simulink model "MPC"  (R2024a)
settings: Solver=ode4  StartTime=0.0  StopTime=5  FixedStep=1e-6  RelTol=1e-3
PreLoadFcn:
  | Rs=0.02;
  | Ls=0.4;
  | Sm=0.2205;
  | p=4;
  | J=0.006;
  | B=0;
  | f=60;
libraries: slpidlib x1
settings Model: Creator=Windows10  LastModifiedBy=anugr
settings SolverCC: AlgebraicLoopSolver=TrustRegion
settings DataIOCC: ReturnWorkspaceOutputs=off
settings DebuggingCC: UnconnectedInputMsg=warning  UnconnectedOutputMsg=warning  UnconnectedLineMsg=warning  UnderSpecifiedDimensionMsg=warning
settings ModelReferenceCC: EnableRefExpFcnMdlSchedulingChecks=on
settings RTWCC: GPUComputeCapability=3.5

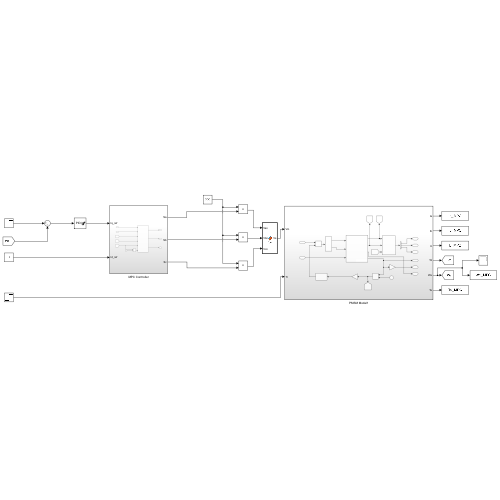
[thumbnail: Simulink's stored preview of the top-level diagram]
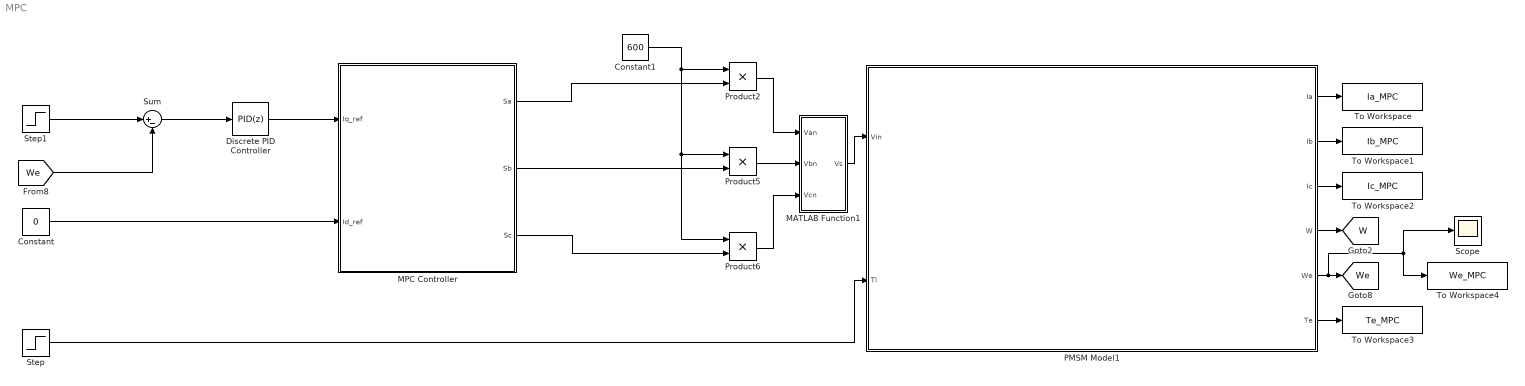
== system MPC ==
  Constant : Constant  Value=0
  Constant1 : Constant  Value=600
  Discrete PID Controller : slpidlib/PID Controller  Controller=PID  Form=Parallel  TimeDomain=Discrete-time  UseExternalTs=off  SampleTime=-1  IntegratorMethod=Forward Euler  FilterMethod=Forward Euler  ControllerParametersSource=internal  P=10  I=1  UseKiTs=off  D=1  UseExternalDerivativeSource=off  N=100  UseFilter=off  TunerSelectOption=Transfer Function Based (PID Tuner App)  InitialConditionSource=internal  InitialConditionForIntegrator=0  InitialConditionForFilter=0  DifferentiatorICPrevScaledInput=0  ExternalReset=none  TrackingMode=off  Kt=1  LimitOutput=on  SatLimitsSource=internal  UpperSaturationLimit=90  LowerSaturationLimit=-90  LinearizeAsGain=on  AntiWindupMode=clamping  Kb=1  LimitIntegrator=off  UpperIntegratorSaturationLimit=inf  LowerIntegratorSaturationLimit=-inf  POutMin=[]  POutMax=[]  IOutMin=[]  IOutMax=[]  DOutMin=[]  DOutMax=[]  NOutMin=[]  NOutMax=[]  SumOutMin=[]  SumOutMax=[]  SaturationOutMin=[]  SaturationOutMax=[]  PParamMin=[]  PParamMax=[]  IParamMin=[]  IParamMax=[]  DParamMin=[]  DParamMax=[]  NParamMin=[]  NParamMax=[]  KbParamMin=[]  KbParamMax=[]  KtParamMin=[]  KtParamMax=[]  KbOutMin=[]  KbOutMax=[]  KtOutMin=[]  KtOutMax=[]  IntegratorOutMin=[]  IntegratorOutMax=[]  FilterOutMin=[]  FilterOutMax=[]  SumI1OutMin=[]  SumI1OutMax=[]  SumI2OutMin=[]  SumI2OutMax=[]  SumI3OutMin=[]  SumI3OutMax=[]  SumI4OutMin=[]  SumI4OutMax=[]  SumDOutMin=[]  SumDOutMax=[]  DifferentiatorOutMin=[]  DifferentiatorOutMax=[]  FilterDiffOutCoefMin=[]  FilterDiffOutCoefMax=[]  ReciprocalOutMin=[]  ReciprocalOutMax=[]  SumDenOutMin=[]  SumDenOutMax=[]  SumNumOutMin=[]  SumNumOutMax=[]  DivideOutMin=[]  DivideOutMax=[]  UdiffTsProdOutMin=[]  UdiffTsProdOutMax=[]  NTsProdOutMin=[]  NTsProdOutMax=[]  UintegralTsProdOutMin=[]  UintegralTsProdOutMax=[]  UngainTsProdOutMin=[]  UngainTsProdOutMax=[]  ClampingZeroOutDataTypeStr=Inherit: Inherit via back propagation  ClampingZeroOutMin=[]  ClampingZeroOutMax=[]  FilterDenConstantOutDataTypeStr=Inherit: Inherit via back propagation  FilterDenConstantOutMin=[]  FilterDenConstantOutMax=[]  PCopyOutDataTypeStr=Inherit: Inherit via back propagation  PCopyOutMin=[]  PCopyOutMax=[]  NCopyOutDataTypeStr=Inherit: Inherit via back propagation  NCopyOutMin=[]  NCopyOutMax=[]  IntegratorContinuousStateAttributes=''  IntegratorStateMustResolveToSignalObject=off  IntegratorRTWStateStorageClass=Auto  FilterContinuousStateAttributes=''  FilterStateMustResolveToSignalObject=off  FilterRTWStateStorageClass=Auto  ParallelPVariant=InternalParameters  IdealPVariant=Disabled  IVariant=InternalParameters  DVariant=InternalParameters  IntegratorVariant=Discrete  SatVariant=Enabled  AWVariant=DiscClampingParallel  PCopyVariant=Disabled  TRVariant=Disabled  FdbkBlocksVariant=Forward  IdealPFdbkVariant=Disabled  SatFdbkVariant=Disabled  DerivativeFilterVariant=Differentiator  NVariant=Passthrough  NCopyVariant=Disabled_SignalSpec  FilterICVariant=InternalICsDifferentiator  IntegratorICVariant=InternalICs  ExternalResetVariant=Disabled  TRSumVariant=Passthrough  SumFdbkVariant=Disabled  SumVariant=Sum_PID  TsampFilterVariant=InternalTs  TsampNgainVariant=Passthrough  TsampIntegralVariant=Disabled_SignalSpec  ExternalSaturationOutDataTypeStr=Inherit: Same as second input  DerivativeSourceVariant=ErrorSignal
  MATLAB Function1 : MATLAB Function  TreatAsAtomicUnit=on
  MPC Controller : Subsystem
  PMSM Model1 : Subsystem
  Product2 : Product
  Product5 : Product
  Product6 : Product
  Scope : Scope
  Step : Step  Time=2.5  After=5  SampleTime=0
  Step1 : Step  Time=2  Before=300  After=800  SampleTime=0
  Sum : Sum  Inputs=|+-
  To Workspace : ToWorkspace  VariableName=Ia_MPC  SaveFormat=Timeseries  SampleTime=-1
  To Workspace1 : ToWorkspace  VariableName=Ib_MPC  SaveFormat=Timeseries  SampleTime=-1
  To Workspace2 : ToWorkspace  VariableName=Ic_MPC  SaveFormat=Timeseries  SampleTime=-1
  To Workspace3 : ToWorkspace  VariableName=Te_MPC  SaveFormat=Timeseries  SampleTime=-1
  To Workspace4 : ToWorkspace  VariableName=We_MPC  SaveFormat=Timeseries  SampleTime=-1
  tag scope: W=global, We=global
  wires:
  Sum/1 -> Discrete PID Controller/1
  [We] -> Sum/2
  Step1/1 -> Sum/1
  Discrete PID Controller/1 -> MPC Controller/1(Iq_ref)
  Step/1 -> PMSM Model1/2(Tl)
  Constant/1 -> MPC Controller/2(Id_ref)
  PMSM Model1/1(Ia) -> To Workspace/1
  PMSM Model1/2(Ib) -> To Workspace1/1
  MATLAB Function1/1(Vs) -> PMSM Model1/1(Vin)
  Constant1/1 -> Product5/1, Product6/1, Product2/1
  Product6/1 -> MATLAB Function1/3(Vcn)
  Product2/1 -> MATLAB Function1/1(Van)
  PMSM Model1/5(We) -> Scope/1, To Workspace4/1, [We]
  PMSM Model1/3(Ic) -> To Workspace2/1
  PMSM Model1/4(W) -> [W]
  Product5/1 -> MATLAB Function1/2(Vbn)
  PMSM Model1/6(Te) -> To Workspace3/1
  MPC Controller/3(Sc) -> Product6/2
  MPC Controller/1(Sa) -> Product2/2
  MPC Controller/2(Sb) -> Product5/2

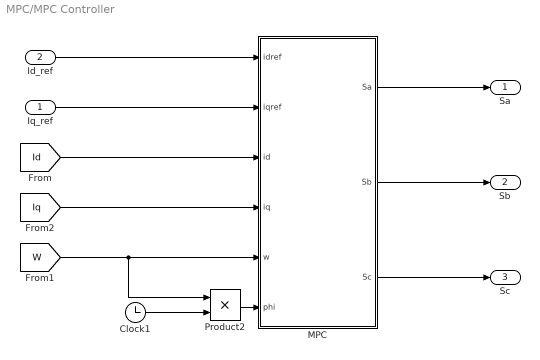
== system MPC/MPC Controller ==
  Iq_ref : Inport
  Id_ref : Inport  Port=2
  Clock1 : Clock
  MPC : MATLAB Function  TreatAsAtomicUnit=on
  Product2 : Product
  Sa : Outport
  Sb : Outport  Port=2
  Sc : Outport  Port=3
  wires:
  [Iq] -> MPC/4(iq)
  [W] -> MPC/5(w), Product2/1
  MPC/3(Sc) -> Sc/1
  [Id] -> MPC/3(id)
  Id_ref/1 -> MPC/1(idref)
  Iq_ref/1 -> MPC/2(iqref)
  Product2/1 -> MPC/6(phi)
  Clock1/1 -> Product2/2
  MPC/2(Sb) -> Sb/1
  MPC/1(Sa) -> Sa/1

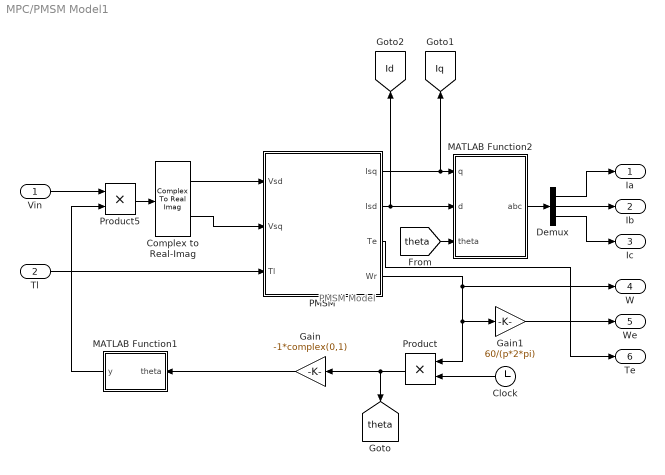
== system MPC/PMSM Model1 ==
  note: PMSM Model
  Vin : Inport
  Tl : Inport  Port=2
  Clock : Clock
  Complex to Real-Imag : ComplexToRealImag
  Demux : Demux  Outputs=3
  Gain : Gain  Gain=-1*complex(0,1)
  Gain1 : Gain  Gain=60/(p*2*pi)
  MATLAB Function1 : MATLAB Function  TreatAsAtomicUnit=on
  MATLAB Function2 : MATLAB Function  TreatAsAtomicUnit=on
  PMSM : Subsystem
  Product : Product
  Product5 : Product
  Ia : Outport
  Ib : Outport  Port=2
  Ic : Outport  Port=3
  W : Outport  Port=4
  We : Outport  Port=5
  Te : Outport  Port=6
  tag scope: Id=global, Iq=global, theta=global
  wires:
  Tl/1 -> PMSM/3(Tl)
  PMSM/4(Wr) -> W/1, Gain1/1, Product/1
  Product/1 -> Gain/1, [theta]
  Demux/3 -> Ic/1
  Clock/1 -> Product/2
  PMSM/1(Isq) -> [Iq], MATLAB Function2/1(q)
  MATLAB Function1/1(y) -> Product5/2
  Complex to Real-Imag/1 -> PMSM/1(Vsd)
  PMSM/3(Te) -> Te/1
  PMSM/2(Isd) -> MATLAB Function2/2(d), [Id]
  Complex to Real-Imag/2 -> PMSM/2(Vsq)
  Product5/1 -> Complex to Real-Imag/1
  Gain/1 -> MATLAB Function1/1(theta)
  Demux/1 -> Ia/1
  MATLAB Function2/1(abc) -> Demux/1
  Vin/1 -> Product5/1
  Gain1/1 -> We/1
  Demux/2 -> Ib/1
  [theta] -> MATLAB Function2/3(theta)

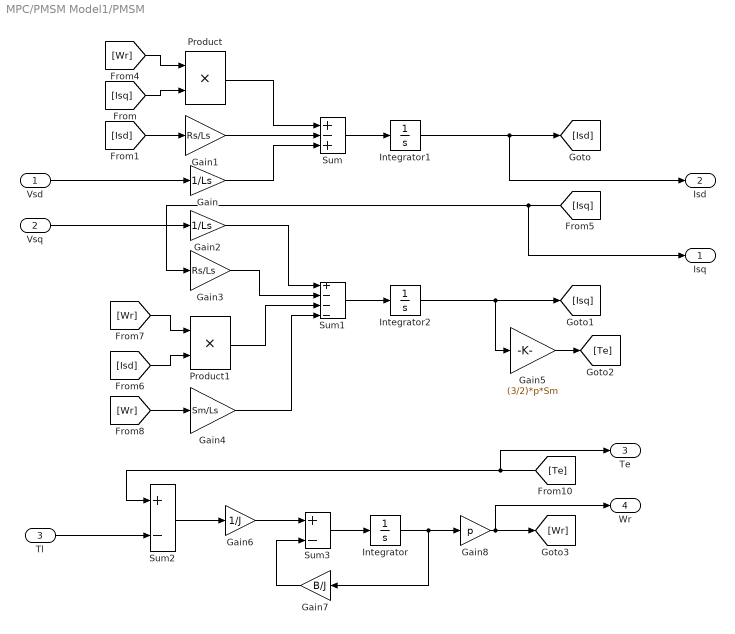
== system MPC/PMSM Model1/PMSM ==
  Vsd : Inport
  Vsq : Inport  Port=2
  Tl : Inport  Port=3
  Gain : Gain  Gain=1/Ls
  Gain1 : Gain  Gain=Rs/Ls
  Gain2 : Gain  Gain=1/Ls
  Gain3 : Gain  Gain=Rs/Ls
  Gain4 : Gain  Gain=Sm/Ls
  Gain5 : Gain  Gain=(3/2)*p*Sm
  Gain6 : Gain  Gain=1/J
  Gain7 : Gain  Gain=B/J
  Gain8 : Gain  Gain=p
  Integrator : Integrator
  Integrator1 : Integrator
  Integrator2 : Integrator
  Product : Product
  Product1 : Product
  Sum : Sum  Inputs=+-+
  Sum1 : Sum  Inputs=+---
  Sum2 : Sum  Inputs=+-
  Sum3 : Sum  Inputs=+-
  Isq : Outport
  Isd : Outport  Port=2
  Te : Outport  Port=3
  Wr : Outport  Port=4
  wires:
  Gain5/1 -> [Te]
  [Wr] -> Gain4/1
  [Isq] -> Isq/1, Gain3/1
  [Te] -> Te/1, Sum2/1
  Integrator2/1 -> Gain5/1, [Isq]
  Gain6/1 -> Sum3/1
  Sum1/1 -> Integrator2/1
  Gain/1 -> Sum/3
  Integrator/1 -> Gain8/1, Gain7/1
  Tl/1 -> Sum2/2
  Gain8/1 -> Wr/1, [Wr]
  Gain2/1 -> Sum1/1
  Sum3/1 -> Integrator/1
  Vsd/1 -> Gain/1
  Sum2/1 -> Gain6/1
  [Isd] -> Product1/2
  Gain7/1 -> Sum3/2
  Gain3/1 -> Sum1/2
  Gain4/1 -> Sum1/4
  [Wr] -> Product/1
  [Isq] -> Product/2
  Product1/1 -> Sum1/3
  [Wr] -> Product1/1
  Product/1 -> Sum/1
  Gain1/1 -> Sum/2
  [Isd] -> Gain1/1
  Sum/1 -> Integrator1/1
  Vsq/1 -> Gain2/1
  Integrator1/1 -> Isd/1, [Isd]

== matlab function MPC/MPC Controller/MPC ==
  settings: updateMethod=DISCRETE
  data: idref input; Sa output; iqref input; id input; iq input; w input; Sb output; Sc output; phi input
function [Sa, Sb, Sc] = mpc(idref, iqref, id, iq, w,phi) 
    %% Initialisation 
    R = 0.02;
    Ls = 0.4;
    Vdc = 400;
    Lambda_f = 0.2205;
    Ts = 1e-6;
    imax=80;
    p=4;
    cost=1e14; 
    persistent state; 
    if isempty(state) 
        state = 1; 
    end
    S = [0 0 0; 1 0 0; 1 1 0; 0 1 0; 0 1 1; 0 0 1; 1 0 1; 1 1 1]; 
    for i=1:8
    ud = Vdc*(2/3)*(S(i,1)*cos(phi) + S(i,2)*cos(phi-2*pi/3) + S(i,3)*cos(phi + 2*pi/3)); 
    uq = Vdc*(2/3)* (-S(i,1) *sin(phi) - S(i,2)*sin(phi- 2*pi/3) - S(i,3)*sin(phi + 2*pi/3));
    id1 = ((1 -(R*Ts)/Ls)*id) + ((Ts*ud)/Ls) + (w*Ts*iq) ; 
    iq1 = ((1 - (R*Ts)/Ls)*iq) + ((Ts*uq)/Ls) - ((w*Ts*id)) - (((w*Ts*Lambda_f)/Ls)); 
    f = 0; 
    if abs(id1) > imax || abs(iq1) > imax 
        f = 1e14; 
    end
    current_cost=(idref-id1)^2 + (iqref-iq1)^2 +f; 
    if(current_cost<cost) 
        state=i;
        cost=current_cost;
    end
          
    end
    Sa = S(state,1);
    Sb = S(state,2); 
    Sc = S(state,3);
end

== matlab function MPC/MATLAB Function1 ==
  data: Van input; Vs output; Vbn input; Vcn input
function Vs = fcn(Van,Vbn,Vcn)

a=complex(cos(2*pi/3),sin(2*pi/3)); 
Vs =(2/3)*(Van+(a*Vbn)+((a^2)*Vcn)) ;

== matlab function MPC/PMSM Model1/MATLAB Function1 ==
  data: theta input; y output
function y = fcn(theta)

y = exp((theta));

== matlab function MPC/PMSM Model1/MATLAB Function2 ==
  data: q input; d input; abc output; theta input
function abc = dq_to_abc(q, d, theta)
    % Inputs:
    % d, q   : DQ components
    % theta  : Electrical angle in radians

    % Transformation matrix
    T = [cos(theta), -sin(theta), 1; 
         cos(theta - 2*pi/3), -sin(theta - 2*pi/3), 1; 
         cos(theta + 2*pi/3), -sin(theta + 2*pi/3), 1];

    % Calculate abc components
    abc = (2/3) * T * [d; q; 0];
end
